simulink model "thermalResistanceNetworkV3"  (R2021b)
settings: Solver=VariableStepAuto  StartTime=0.0  StopTime=numSec  RelTol=1e-3
undefined symbols (not defined in the file): A_rad, A_solararray_face, m_45bracket, m_XRD, Q_PH
libraries: fl_lib x170, nesl_utility x39
(part 2 of 2)

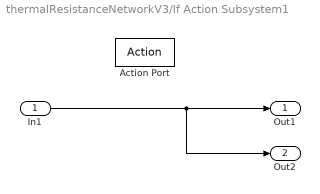
== system thermalResistanceNetworkV3/If Action Subsystem1 ==
  In1 : Inport
  Action Port : ActionPort  ActionPortLabel=if(u1 > 288.5 | u1<278.15)
  Out1 : Outport
  Out2 : Outport  Port=2
  wires:
  In1/1 -> Out2/1, Out1/1

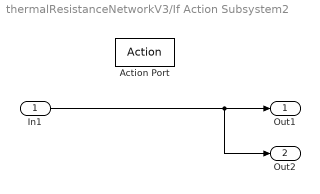
== system thermalResistanceNetworkV3/If Action Subsystem2 ==
  In1 : Inport
  Action Port : ActionPort  ActionPortLabel=if(u1 < 283.15)
  Out1 : Outport
  Out2 : Outport  Port=2
  wires:
  In1/1 -> Out1/1, Out2/1

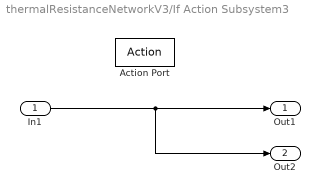
== system thermalResistanceNetworkV3/If Action Subsystem3 ==
  In1 : Inport
  Action Port : ActionPort  ActionPortLabel=if(u1 > 308.5 | u1<278.15)
  Out1 : Outport
  Out2 : Outport  Port=2
  wires:
  In1/1 -> Out2/1, Out1/1

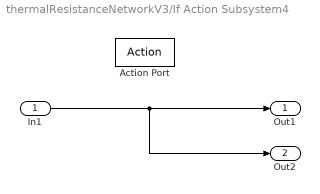
== system thermalResistanceNetworkV3/If Action Subsystem4 ==
  In1 : Inport
  Action Port : ActionPort  ActionPortLabel=else
  Out1 : Outport
  Out2 : Outport  Port=2
  wires:
  In1/1 -> Out2/1, Out1/1

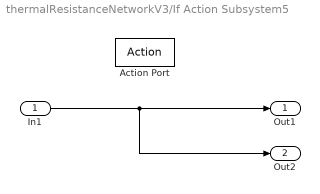
== system thermalResistanceNetworkV3/If Action Subsystem5 ==
  In1 : Inport
  Action Port : ActionPort  ActionPortLabel=else
  Out1 : Outport
  Out2 : Outport  Port=2
  wires:
  In1/1 -> Out2/1, Out1/1

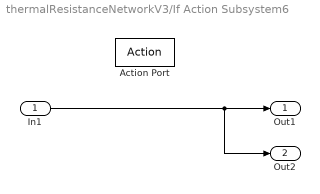
== system thermalResistanceNetworkV3/If Action Subsystem6 ==
  In1 : Inport
  Action Port : ActionPort  ActionPortLabel=if(u1 < 273.15)
  Out1 : Outport
  Out2 : Outport  Port=2
  wires:
  In1/1 -> Out2/1, Out1/1

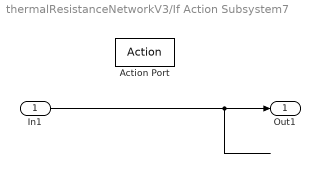
== system thermalResistanceNetworkV3/If Action Subsystem7 ==
  In1 : Inport
  Action Port : ActionPort  ActionPortLabel=if(u1 < 288.15)
  Out1 : Outport
  wires:
  In1/1 -> Out1/1
